simulink model "PowerSupplySimulation5RELoad4"  (R2015b)
settings: Solver=ode23t  StartTime=0.0  StopTime=20*360e-6  MaxStep=1e-7  MinStep=1e-9  RelTol=1e-3
values from neighbouring files (symbols this model uses):
  Ac = 1/(evalfr(G_ss, wcross)*evalfr(Gc1, wcross)*evalfr(Gc2, wcross))    [CurrentSourceController.m]    (also in VoltageSourceController.m; master_conv.m)
  c2_val = 1e-6    (= 1e-06)    [VoltageSourceController.m]    (also in master_conv.m = 2.5e-08)
  delay_load = t1    (= 5.4e-06)    [master_conv.m]
  duty_inv = 100 - duty    (= 90)    [master_conv.m]
  duty_load = (t2-t1)/T_mach*100    (= 7)    [master_conv.m]
  Eg = 30    [RippleCalculations.m]    (also in master_conv.m)
  I_ref = 10    [RippleCalculations.m]    (also in master_conv.m)
  l1_val = 480e-8    (= 4.8e-06)    [CurrentSourceController.m]    (also in master_conv.m = 5.09090909091e-05)
  l2_val = 0.01e-6    (= 1e-08)    [VoltageSourceController.m]    (also in master_conv.m = 1.81818181818e-05)
  r_val = 1    [CurrentSourceController.m]    (also in master_conv.m)
  rc2_val = 0.0001    [VoltageSourceController.m]    (also in master_conv.m)
  rl1_val = 0.0002    [CurrentSourceController.m]    (also in master_conv.m)
  rl2_val = 0.0001    [VoltageSourceController.m]    (also in master_conv.m)
  t2 = duty * T_mach / 100    (= 1.8e-05)    [master_conv.m]
  T_mach = 180e-6    (= 0.00018)    [master_conv.m]
  V_ref = 80    [RippleCalculations.m]    (also in VoltageSourceController.m; master_conv.m = 100)
  Vd_val = 110    [CurrentSourceController.m]    (also in VoltageSourceController.m; master_conv.m)
undefined symbols (not defined in the file or in its folder): den_c1, den_c2, num_c1, num_c2
libraries: powerlib x33, powerlib_meascontrol x2
settings Model: Creator=Akshay  LastModifiedBy=Akshay
settings SolverCC: ZeroCrossAlgorithm=Adaptive
settings DataIOCC: SaveFormat=StructureWithTime
settings HardwareCC: ProdWordSize=32  ProdHWDeviceType=Specified

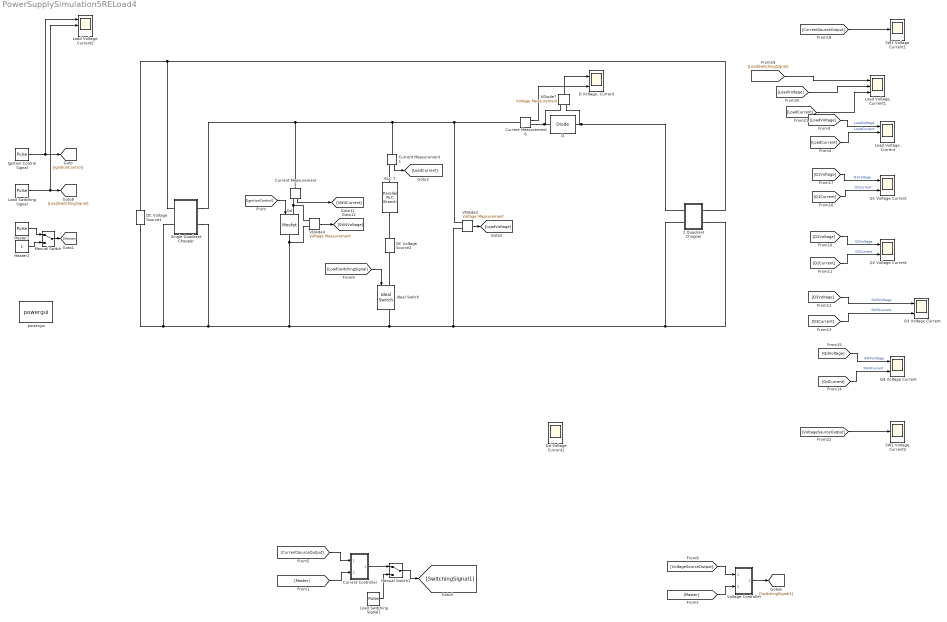
== system PowerSupplySimulation5RELoad4 ==
  " RLC 7" : powerlib/Elements/Parallel RLC Branch  LConnTagsString=a  RConnTagsString=__new0  BranchType=R  Resistance=r_val  Inductance=1e-3  SetiL0=off  InitialCurrent=0  Capacitance=0.1e-6  Setx0=off  InitialVoltage=0  Measurements=None
  2 Quadrant Chopper : Subsystem
  Current Measurement1 : powerlib/Measurements/Current Measurement  PhasorSimulation=off  OutputType=Complex  PSBequivalent=0
  Current Measurement3 : powerlib/Measurements/Current Measurement  PhasorSimulation=off  OutputType=Complex  PSBequivalent=0
  Current Measurement6 : powerlib/Measurements/Current Measurement  PhasorSimulation=off  OutputType=Complex  PSBequivalent=0
  Current Controller : Subsystem
  D : powerlib/Power Electronics/Diode  Ron=0.001  Lon=0  Vf=0.8  IC=0  UseSnubber=off  Rs=500  Cs=250e-9  Measurements=off
  "D Voltage, Current" : Scope  NumInputPorts=2
  DC Voltage Source1 : powerlib/Electrical Sources/DC Voltage Source  Amplitude=Vd_val  Measurements=Voltage
  DC Voltage Source2 : powerlib/Electrical Sources/DC Voltage Source  Amplitude=Eg  Measurements=Voltage
  Ideal Switch : powerlib/Power Electronics/Ideal Switch  Ron=0.001  Lon=0  IC=0  Rs=1e5  Cs=inf  Measurements=on
  Ignition Control Signal : DiscretePulseGenerator  PulseType=Time based  Period=T_mach  PulseWidth=duty_inv  PhaseDelay=t2
  Load Switching Signal : DiscretePulseGenerator  PulseType=Time based  Period=T_mach  PulseWidth=duty_load  PhaseDelay=delay_load
  Load Switching Signal1 : DiscretePulseGenerator  PulseType=Time based  Period=180e-6  PulseWidth=6  PhaseDelay=1.8e-6
  "Load Voltage, Current" : Scope  NumInputPorts=3
  "Load Voltage, Current1" : Scope  NumInputPorts=3
  "Load Voltage, Current2" : Scope  NumInputPorts=3
  Manual Switch : ManualSwitch
  Manual Switch1 : ManualSwitch
  Master1 : DiscretePulseGenerator  PulseType=Time based  Period=180e-6  PulseWidth=6
  Master2 : Constant
  Q1 Voltage Current : Scope  NumInputPorts=2
  Q2 Voltage Current : Scope  NumInputPorts=2
  Q3 Voltage Current : Scope  NumInputPorts=2
  Qd : powerlib/Power Electronics/Mosfet  Ron=0.00001  Lon=0  Rd=0.0000000000001  Vfd=0  IC=0  Rs=1e5  Cs=inf  Measurements=off
  Qd Voltage Current : Scope  NumInputPorts=2
  Qd Voltage Current1 : Scope  NumInputPorts=2
  "SW1 Voltage, Current1" : Scope
  "SW1 Voltage, Current2" : Scope
  Single Quadrant Chopper : Subsystem
  VDiode2 : powerlib/Measurements/Voltage Measurement  PhasorSimulation=off  OutputType=Complex  PSBequivalent=0
  VDiode4 : powerlib/Measurements/Voltage Measurement  PhasorSimulation=off  OutputType=Complex  PSBequivalent=0
  VDiode7 : powerlib/Measurements/Voltage Measurement  PhasorSimulation=off  OutputType=Complex  PSBequivalent=0
  Voltage Controller : Subsystem
  powergui : powerlib/powergui  Priority=1  SimulationMode=Continuous  SolverType=Backward Euler  SampleTime=5e-07  frequency=60  SPID=on  DisableSnubberDevices=off  DisableRonSwitches=off  DisableVfSwitches=off  SwTol=0  DisplayEquations=off  Interpol=off  ExternalGateDelay=off  methode=off  Ts=0  FunctionMessages=off  echomessages=off  HookPort=off  EnableUseOfTLC=off  x0status=zero  frequencyindice=0  Pbase=100e6  ErrMax=1e-4  Iterations=50  UnitsV=kV  UnitsW=MW  buscounter=0  RestoreLinks=warning  ResistiveCurrentMeasurement=off  Frange=[0:2:500]  Ylog=off  Xlog=on  ShowGrid=off  save=off  variable=ZData  structure=ScopeData  ZoomFFT=off  StartTime=0.0  cycles=5  DisplayStyle=2  fundamental=50  FreqAxis=off  MaxFrequency=50000  frequencyindicesteady=1  RmsSteady=1  display=off
  wires:
  Ignition Control Signal/1 -> "Load Voltage, Current2"/1, [IgnitionControl]
  [IgnitionControl] -> Qd/1
  VDiode2/1 -> [LoadVoltage]
  Current Measurement1/1 -> [LoadCurrent]
  [LoadVoltage] -> "Load Voltage, Current"/1  "LoadVoltage"
  [LoadCurrent] -> "Load Voltage, Current"/2  "LoadCurrent"
  Load Switching Signal/1 -> "Load Voltage, Current2"/2, [LoadSwitchingSignal]
  [LoadSwitchingSignal] -> Ideal Switch/1
  Manual Switch/1 -> [Master]
  Master1/1 -> Manual Switch/1
  Master2/1 -> Manual Switch/2
  Current Measurement3/1 -> [SW4Current]
  VDiode4/1 -> [SW4Voltage]
  [Q2Voltage] -> Q2 Voltage Current/1  "Q2Voltage"
  [Q2Current] -> Q2 Voltage Current/2  "Q2Current"
  [Q3Voltage] -> Q3 Voltage Current/1  "SW3Voltage"
  [Q3Current] -> Q3 Voltage Current/2  "SW3Current"
  [Q1Voltage] -> Q1 Voltage Current/1  "Q1Voltage"
  [Q1Current] -> Q1 Voltage Current/2  "Q1Current"
  [QdVoltage] -> Qd Voltage Current/1  "SW4Voltage"
  [QdCurrent] -> Qd Voltage Current/2  "SW4Current"
  Current Measurement6/1 -> "D Voltage, Current"/2
  VDiode7/1 -> "D Voltage, Current"/1
  [LoadSwitchingSignal] -> "Load Voltage, Current1"/1
  [LoadVoltage] -> "Load Voltage, Current1"/2
  [LoadCurrent] -> "Load Voltage, Current1"/3
  [VoltageSourceOutput] -> "SW1 Voltage, Current2"/1
  [CurrentSourceOutput] -> "SW1 Voltage, Current1"/1
  [VoltageSourceOutput] -> Voltage Controller/1(In1)
  [Master] -> Voltage Controller/2(In2)
  Voltage Controller/1(Out1) -> [SwitchingSignal2]
  [CurrentSourceOutput] -> Current Controller/1(In1)
  [Master] -> Current Controller/2(In2)
  Current Controller/1(Out1) -> Manual Switch1/1
  Manual Switch1/1 -> [SwitchingSignal1]
  Load Switching Signal1/1 -> Manual Switch1/2
  connections:
  VDiode7/LConn2 -- 2 Quadrant Chopper/LConn1 -- D/RConn1
  Single Quadrant Chopper/RConn1 -- VDiode2/LConn1 -- Current Measurement6/LConn1 -- Current Measurement1/LConn1 -- Current Measurement3/LConn1
  Current Measurement3/RConn1 -- VDiode4/LConn1 -- Qd/LConn1
  Current Measurement6/RConn1 -- VDiode7/LConn1 -- D/LConn1
  DC Voltage Source1/RConn1 -- Single Quadrant Chopper/LConn1 -- 2 Quadrant Chopper/RConn1
  Qd/RConn1 -- VDiode4/LConn2 -- Single Quadrant Chopper/RConn2 -- DC Voltage Source1/LConn1 -- Single Quadrant Chopper/LConn2 -- 2 Quadrant Chopper/RConn2 -- 2 Quadrant Chopper/LConn2 -- VDiode2/LConn2 -- Ideal Switch/RConn1
  Ideal Switch/LConn1 -- DC Voltage Source2/LConn1
  DC Voltage Source2/RConn1 -- " RLC 7"/RConn1
  Current Measurement1/RConn1 -- " RLC 7"/LConn1

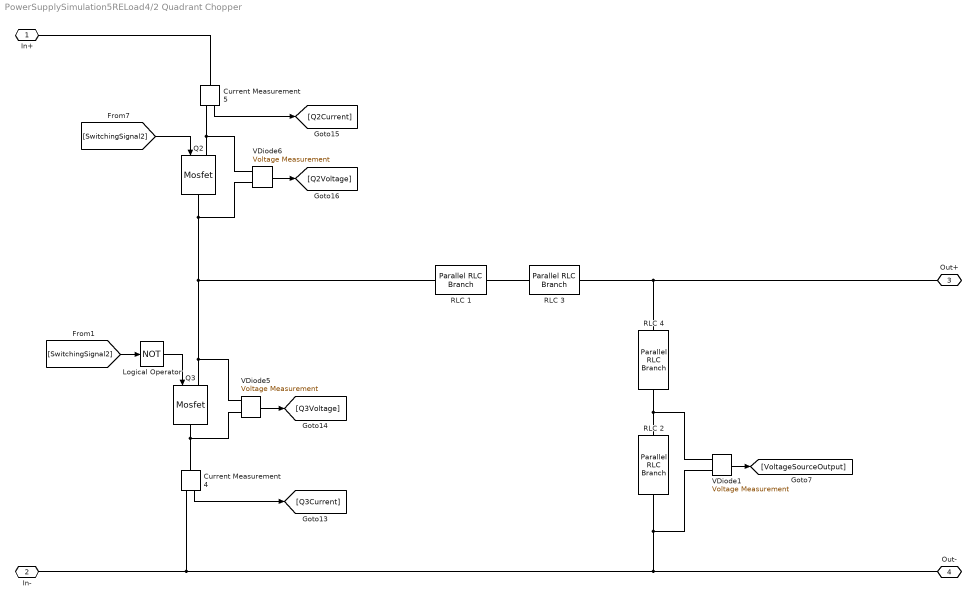
== system PowerSupplySimulation5RELoad4/2 Quadrant Chopper ==
  " RLC 1" : powerlib/Elements/Parallel RLC Branch  LConnTagsString=a  RConnTagsString=__new0  BranchType=R  Resistance=rl2_val  Inductance=5e-6  SetiL0=off  InitialCurrent=0  Capacitance=0.3e-6  Setx0=off  InitialVoltage=0  Measurements=None
  " RLC 2" : powerlib/Elements/Parallel RLC Branch  LConnTagsString=a  RConnTagsString=__new0  BranchType=C  Resistance=1  Inductance=1e-3  SetiL0=off  InitialCurrent=0  Capacitance=c2_val  Setx0=off  InitialVoltage=50  Measurements=None
  " RLC 3" : powerlib/Elements/Parallel RLC Branch  LConnTagsString=a  RConnTagsString=__new0  BranchType=L  Resistance=50  Inductance=l2_val  SetiL0=off  InitialCurrent=0  Capacitance=0.3e-6  Setx0=off  InitialVoltage=0  Measurements=None
  " RLC 4" : powerlib/Elements/Parallel RLC Branch  LConnTagsString=a  RConnTagsString=__new0  BranchType=R  Resistance=rc2_val  Inductance=1e-3  SetiL0=off  InitialCurrent=0  Capacitance=0.1e-6  Setx0=off  InitialVoltage=0  Measurements=None
  Current Measurement4 : powerlib/Measurements/Current Measurement  PhasorSimulation=off  OutputType=Complex  PSBequivalent=0
  Current Measurement5 : powerlib/Measurements/Current Measurement  PhasorSimulation=off  OutputType=Complex  PSBequivalent=0
  Logical Operator : Logic  Operator=NOT  AllPortsSameDT=off  OutDataTypeStr=boolean
  Q2 : powerlib/Power Electronics/Mosfet  Ron=0.00001  Lon=0  Rd=0.0000000000001  Vfd=0  IC=0  Rs=1e5  Cs=inf  Measurements=off
  Q3 : powerlib/Power Electronics/Mosfet  Ron=0.00001  Lon=0  Rd=0.0000000000001  Vfd=0  IC=0  Rs=1e5  Cs=inf  Measurements=off
  VDiode1 : powerlib/Measurements/Voltage Measurement  PhasorSimulation=off  OutputType=Complex  PSBequivalent=0
  VDiode5 : powerlib/Measurements/Voltage Measurement  PhasorSimulation=off  OutputType=Complex  PSBequivalent=0
  VDiode6 : powerlib/Measurements/Voltage Measurement  PhasorSimulation=off  OutputType=Complex  PSBequivalent=0
  In+ : PMIOPort  Port=1  Side=Right
  In- : PMIOPort  Port=2  Side=Right
  Out+ : PMIOPort  Port=3  Side=Left
  Out- : PMIOPort  Port=4  Side=Left
  wires:
  VDiode1/1 -> [VoltageSourceOutput]
  VDiode6/1 -> [Q2Voltage]
  Current Measurement5/1 -> [Q2Current]
  [SwitchingSignal2] -> Q2/1
  Logical Operator/1 -> Q3/1
  VDiode5/1 -> [Q3Voltage]
  Current Measurement4/1 -> [Q3Current]
  [SwitchingSignal2] -> Logical Operator/1
  connections:
  " RLC 2"/LConn1 -- VDiode1/LConn1 -- " RLC 4"/RConn1
  " RLC 1"/RConn1 -- " RLC 3"/LConn1
  Current Measurement4/RConn1 -- In-/RConn1 -- Out-/RConn1 -- " RLC 2"/RConn1 -- VDiode1/LConn2
  Current Measurement5/RConn1 -- VDiode6/LConn1 -- Q2/LConn1
  Q2/RConn1 -- VDiode6/LConn2 -- " RLC 1"/LConn1 -- VDiode5/LConn1 -- Q3/LConn1
  Q3/RConn1 -- Current Measurement4/LConn1 -- VDiode5/LConn2
  " RLC 3"/RConn1 -- Out+/RConn1 -- " RLC 4"/LConn1
  In+/RConn1 -- Current Measurement5/LConn1

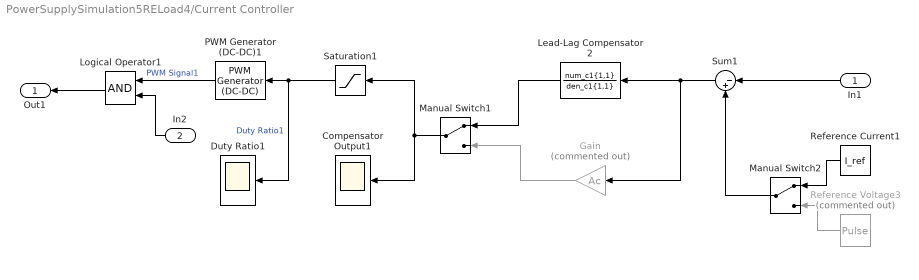
== system PowerSupplySimulation5RELoad4/Current Controller ==
  In1 : Inport
  In2 : Inport  Port=2
  Compensator Output1 : Scope
  Duty Ratio1 : Scope
  Gain : Gain  Commented=on  Gain=Ac
  Lead-Lag Compensator2 : TransferFcn  Numerator=num_c1{1,1}  Denominator=den_c1{1,1}
  Logical Operator1 : Logic  AllPortsSameDT=off  OutDataTypeStr=boolean
  Manual Switch1 : ManualSwitch
  Manual Switch2 : ManualSwitch
  PWM Generator (DC-DC)1 : powerlib_meascontrol/Pulse & Signal Generators/PWM Generator (DC-DC)  Fsw=f_sw  Ts=0
  Reference Current1 : Constant  Value=I_ref
  Reference Voltage3 : DiscretePulseGenerator  Commented=on  PulseType=Time based  Amplitude=70  Period=180e-6  PulseWidth=6
  Saturation1 : Saturate  UpperLimit=1  LowerLimit=0  ZeroCross=off
  Sum1 : Sum  Inputs=|-+
  Out1 : Outport
  wires:
  In2/1 -> Logical Operator1/2
  Logical Operator1/1 -> Out1/1
  Lead-Lag Compensator2/1 -> Manual Switch1/1
  Saturation1/1 -> Duty Ratio1/1, PWM Generator (DC-DC)1/1  "Duty Ratio1"
  In1/1 -> Sum1/1
  PWM Generator (DC-DC)1/1 -> Logical Operator1/1  "PWM Signal1"
  Manual Switch2/1 -> Sum1/2
  Reference Voltage3/1 -> Manual Switch2/2
  Manual Switch1/1 -> Compensator Output1/1, Saturation1/1
  Sum1/1 -> Gain/1, Lead-Lag Compensator2/1
  Reference Current1/1 -> Manual Switch2/1
  Gain/1 -> Manual Switch1/2

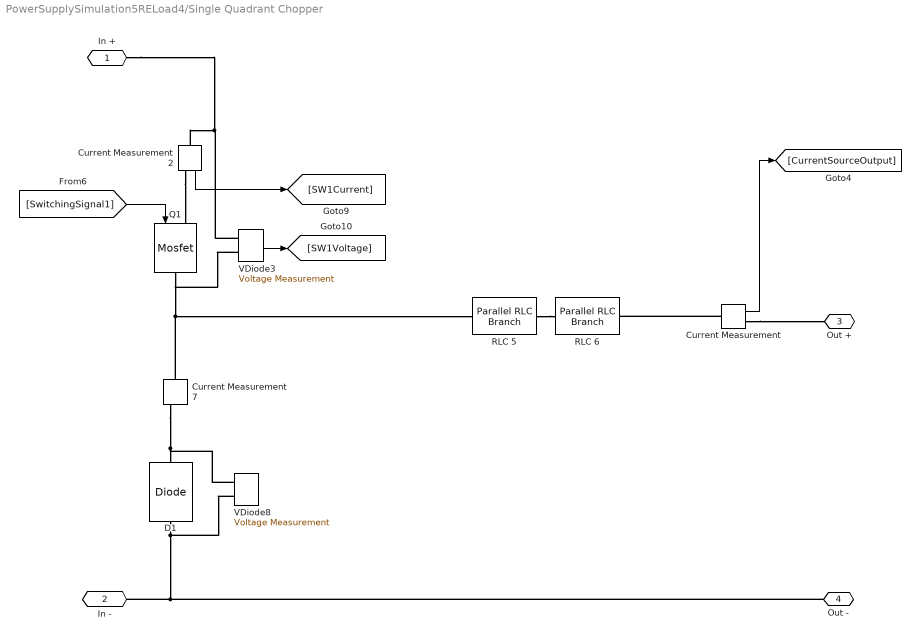
== system PowerSupplySimulation5RELoad4/Single Quadrant Chopper ==
  " RLC 5" : powerlib/Elements/Parallel RLC Branch  LConnTagsString=a  RConnTagsString=__new0  BranchType=R  Resistance=rl1_val  Inductance=5e-6  SetiL0=off  InitialCurrent=0  Capacitance=0.3e-6  Setx0=off  InitialVoltage=0  Measurements=None
  " RLC 6" : powerlib/Elements/Parallel RLC Branch  LConnTagsString=a  RConnTagsString=__new0  BranchType=L  Resistance=50  Inductance=l1_val  SetiL0=off  InitialCurrent=100  Capacitance=0.3e-6  Setx0=off  InitialVoltage=0  Measurements=None
  Current Measurement2 : powerlib/Measurements/Current Measurement  PhasorSimulation=off  OutputType=Complex  PSBequivalent=0
  Current Measurement7 : powerlib/Measurements/Current Measurement  PhasorSimulation=off  OutputType=Complex  PSBequivalent=0
  Current Measurement : powerlib/Measurements/Current Measurement  PhasorSimulation=off  OutputType=Complex  PSBequivalent=0
  D1 : powerlib/Power Electronics/Diode  Ron=0.001  Lon=0  Vf=0.8  IC=0  UseSnubber=off  Rs=500  Cs=250e-9  Measurements=off
  Q1 : powerlib/Power Electronics/Mosfet  Ron=0.00001  Lon=0  Rd=0.0000000000001  Vfd=0  IC=0  Rs=1e5  Cs=inf  Measurements=off
  VDiode3 : powerlib/Measurements/Voltage Measurement  PhasorSimulation=off  OutputType=Complex  PSBequivalent=0
  VDiode8 : powerlib/Measurements/Voltage Measurement  PhasorSimulation=off  OutputType=Complex  PSBequivalent=0
  In + : PMIOPort  Port=1  Side=Left
  In - : PMIOPort  Port=2  Side=Left
  Out + : PMIOPort  Port=3  Side=Right
  Out - : PMIOPort  Port=4  Side=Right
  wires:
  VDiode3/1 -> [SW1Voltage]
  [SwitchingSignal1] -> Q1/1
  Current Measurement2/1 -> [SW1Current]
  Current Measurement/1 -> [CurrentSourceOutput]
  connections:
  VDiode3/LConn2 -- Q1/RConn1 -- Current Measurement7/LConn1 -- " RLC 5"/LConn1
  VDiode3/LConn1 -- Current Measurement2/LConn1 -- In +/RConn1
  " RLC 5"/RConn1 -- " RLC 6"/LConn1
  Current Measurement2/RConn1 -- Q1/LConn1
  Current Measurement7/RConn1 -- VDiode8/LConn1 -- D1/RConn1
  VDiode8/LConn2 -- Out -/RConn1 -- In -/RConn1 -- D1/LConn1
  Current Measurement/LConn1 -- " RLC 6"/RConn1
  Current Measurement/RConn1 -- Out +/RConn1

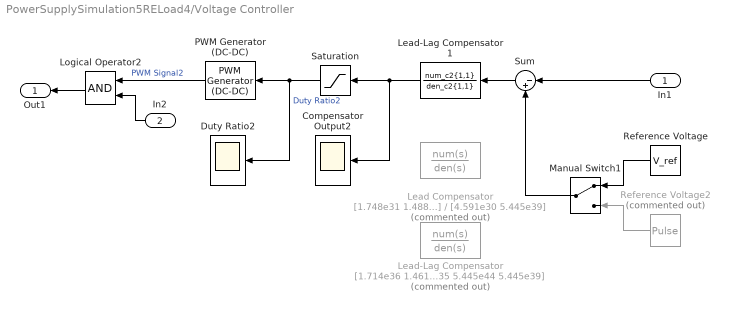
== system PowerSupplySimulation5RELoad4/Voltage Controller ==
  In1 : Inport
  In2 : Inport  Port=2
  Compensator Output2 : Scope
  Duty Ratio2 : Scope
  Lead Compensator : TransferFcn  Commented=on  Numerator=[1.748e31 1.488e39]  Denominator=[4.591e30 5.445e39]
  Lead-Lag Compensator : TransferFcn  Commented=on  Numerator=[1.714e36 1.461e44 1.459e49]  Denominator=[4.591e35 5.445e44 5.445e39]
  Lead-Lag Compensator1 : TransferFcn  Numerator=num_c2{1,1}  Denominator=den_c2{1,1}
  Logical Operator2 : Logic  AllPortsSameDT=off  OutDataTypeStr=boolean
  Manual Switch1 : ManualSwitch
  PWM Generator (DC-DC) : powerlib_meascontrol/Pulse & Signal Generators/PWM Generator (DC-DC)  Fsw=f_sw  Ts=0
  Reference Voltage : Constant  Value=V_ref
  Reference Voltage2 : DiscretePulseGenerator  Commented=on  PulseType=Time based  Amplitude=70  Period=180e-6  PulseWidth=6
  Saturation : Saturate  UpperLimit=1  LowerLimit=0  ZeroCross=off
  Sum : Sum  Inputs=|-+
  Out1 : Outport
  wires:
  Logical Operator2/1 -> Out1/1
  Lead-Lag Compensator1/1 -> Compensator Output2/1, Saturation/1
  Saturation/1 -> Duty Ratio2/1, PWM Generator (DC-DC)/1  "Duty Ratio2"
  Sum/1 -> Lead-Lag Compensator1/1
  In2/1 -> Logical Operator2/2
  PWM Generator (DC-DC)/1 -> Logical Operator2/1  "PWM Signal2"
  In1/1 -> Sum/1
  Reference Voltage/1 -> Manual Switch1/1
  Manual Switch1/1 -> Sum/2
  Reference Voltage2/1 -> Manual Switch1/2
